simulink model "dt_system"  (R2022a)
settings: Solver=ode45  StartTime=0.0  StopTime=tfinal  FixedStep=T  MaxStep=0.01  RelTol=1e-12  AbsTol=1e-12  EnableMultiTasking=on
values from neighbouring files (symbols this model uses):
  Ts = 0.001    [pole_place.m]    (also in pole_zero.m)
libraries: cstblocks x2
settings Model: Creator=cnielsen  LastModifiedBy=urban
settings SolverCC: AutoScaleAbsTol=off  AlgebraicLoopSolver=TrustRegion
settings DataIOCC: SaveFormat=Array  SignalLoggingSaveFormat=ModelDataLogs  SaveOutput=off  SaveTime=off  ReturnWorkspaceOutputs=off  Refine=5
settings OptimizationCC: ExpressionDepthLimit=2147483647  LifeSpan=inf
settings DebuggingCC: UnderspecifiedInitializationDetection=Classic  MergeDetectMultiDrivingBlocksExec=none  SolverPrmCheckMsg=warning  FcnCallInpInsideContextMsg=warning  UnconnectedInputMsg=warning  UnconnectedOutputMsg=warning  UnconnectedLineMsg=warning  StateNameClashWarn=warning  SFUnexpectedBacktrackingDiag=warning  SFNoUnconditionalDefaultTransitionDiag=warning  SFExecutionAtInitializationDiag=none  SFMachineParentedDataDiag=warning  ArithmeticOperatorsInVariantConditions=warning
settings HardwareCC: ProdBitPerPointer=32  ProdBitPerSizeT=32  ProdBitPerPtrDiffT=32  ProdLargestAtomicFloat=None  ProdIntDivRoundTo=Undefined  ProdEndianess=Unspecified  ProdWordSize=32  ProdHWDeviceType=32-bit Generic
settings ModelReferenceCC: PropagateSignalLabelsOutOfModel=off
settings SFSimCC: SimUseLocalCustomCode=off  CustomCodeUndefinedFunction=UseInterfaceOnly
settings RTWCC: RTWUseLocalCustomCode=off
settings CodeAppCC: StateflowObjectComments=on
settings GRTTargetCC: TargetLangStandard=C89/C90 (ANSI)  CombineOutputUpdateFcns=off  GRTInterface=on
settings ConfigComp: CovMetricSettings=dw  CovSaveCumulativeToWorkspaceVar=on  CovSaveSingleToWorkspaceVar=on  CovExternalEMLEnable=off

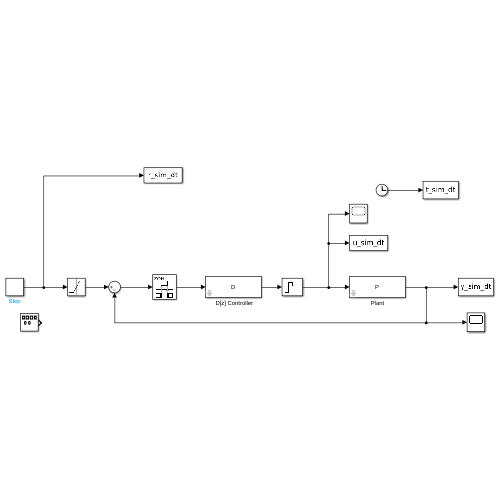
[thumbnail: Simulink's stored preview of the top-level diagram]
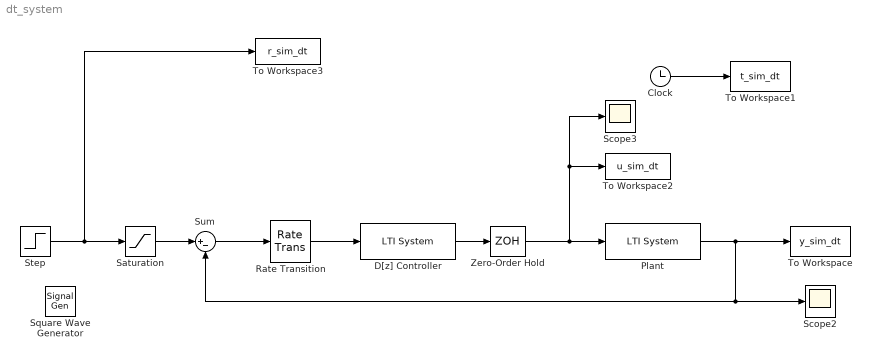
== system dt_system ==
  " D[z] Controller" : cstblocks/LTI System  sys=D  IC=[]
  Clock : Clock
  Plant : cstblocks/LTI System  sys=P  IC=[]
  Rate Transition : RateTransition  OutPortSampleTime=Ts
  Saturation : Saturate  UpperLimit=0.7  LowerLimit=-0.7
  Scope2 : Scope
  Scope3 : Scope
  Square Wave Generator : SignalGenerator  WaveForm=square  Units=rad/sec
  Step : Step  Time=0
  Sum : Sum  Inputs=|+-
  To Workspace : ToWorkspace  VariableName=y_sim_dt  SampleTime=-1
  To Workspace1 : ToWorkspace  VariableName=t_sim_dt  SampleTime=-1
  To Workspace2 : ToWorkspace  VariableName=u_sim_dt
  To Workspace3 : ToWorkspace  VariableName=r_sim_dt
  Zero-Order Hold : ZeroOrderHold  SampleTime=Ts
  wires:
  Clock/1 -> To Workspace1/1
  Plant/1 -> To Workspace/1, Sum/2, Scope2/1
  " D[z] Controller"/1 -> Zero-Order Hold/1
  Sum/1 -> Rate Transition/1
  Rate Transition/1 -> " D[z] Controller"/1
  Zero-Order Hold/1 -> Plant/1, To Workspace2/1, Scope3/1
  Saturation/1 -> Sum/1
  Step/1 -> To Workspace3/1, Saturation/1
